simulink model "ENV"  (R2024b)
settings: Solver=FixedStepDiscrete  StartTime=0.0  StopTime=1  FixedStep=0.001  RelTol=1e-3  EnableMultiTasking=on
libraries: stm32blockslib x92, canmsglib x40, simulink x7, stm32f4xxblockslib x6
(part 2 of 5)

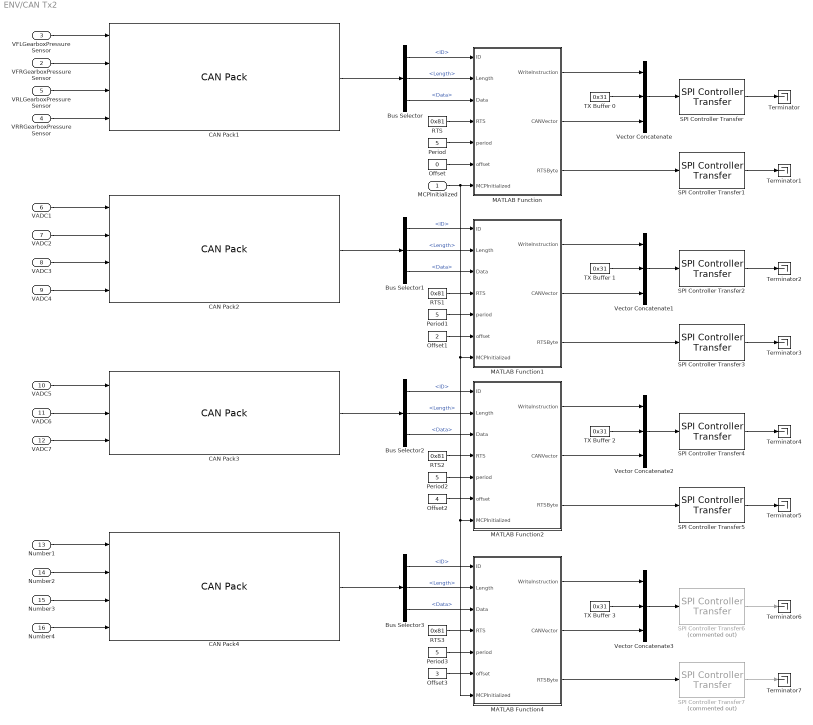
== system ENV/CAN Tx2 ==
  MCPInitialized : Inport
  VFRGearboxPressureSensor : Inport  Port=2
  VFLGearboxPressureSensor : Inport  Port=3
  VRRGearboxPressureSensor : Inport  Port=4
  VRLGearboxPressureSensor : Inport  Port=5
  VADC1 : Inport  Port=6
  VADC2 : Inport  Port=7
  VADC3 : Inport  Port=8
  VADC4 : Inport  Port=9
  VADC5 : Inport  Port=10
  VADC6 : Inport  Port=11
  VADC7 : Inport  Port=12
  Number1 : Inport  Port=13
  Number2 : Inport  Port=14
  Number3 : Inport  Port=15
  Number4 : Inport  Port=16
  Bus Selector{,1..3} (4 alike) : BusSelector  OutputSignals=ID,Length,Data
  CAN Pack1 : canmsglib/CAN Pack  CANdbFile=C:\Users\oxbro\Documents\STM32CustomProjects\PDUSTM32\ADCTest.dbc  MsgList=GearboxPressures  MsgName=GearboxPressures  MsgIDType=Standard (11-bit identifier)  MsgIdentifier=105  CANIDInput=off  MsgLength=8  Remote=off  ApplyMinMax=off  BusOutput=on  SignalInfo={'VFLGearboxPressureSensor','0','12','LE','unsigned','Standard','0','0.0012211','0','0','5.0004';'VFRGearboxPressureSensor','16','12','LE','unsigned','Standard','0','0.0012211','0','0','5.0004';'VRLGearboxPressureSensor','32','12','LE','unsigned','Standard','0','0.0012211','0','0','5.0004';'VRRGearboxPressureSensor','48','12','LE','unsigned','Standard','0','0.0012211','0','0','5.0004'}
      settings: LibrarySourceBlock=stmutilitieslib/CAN Pack  DataFormat=CANdb specified signals
  CAN Pack2 : canmsglib/CAN Pack  CANdbFile=C:\Users\oxbro\Documents\STM32CustomProjects\PDUSTM32\ADCTest.dbc  MsgList=ADCs1  MsgName=ADCs1  MsgIDType=Standard (11-bit identifier)  MsgIdentifier=5  CANIDInput=off  MsgLength=8  Remote=off  ApplyMinMax=off  BusOutput=on  SignalInfo={'VADC1','0','16','LE','unsigned','Standard','0','5.04e-05','0','0','3.303';'VADC2','16','16','LE','unsigned','Standard','0','5.04e-05','0','0','3.303';'VADC3','32','16','LE','unsigned','Standard','0','5.04e-05','0','0','3.303';'VADC4','48','16','LE','unsigned','Standard','0','5.04e-05','0','0','3.303'}
      settings: LibrarySourceBlock=stmutilitieslib/CAN Pack  DataFormat=CANdb specified signals
  CAN Pack3 : canmsglib/CAN Pack  CANdbFile=C:\Users\oxbro\Documents\STM32CustomProjects\PDUSTM32\ADCTest.dbc  MsgList=ADCs2  MsgName=ADCs2  MsgIDType=Standard (11-bit identifier)  MsgIdentifier=66  CANIDInput=off  MsgLength=6  Remote=off  ApplyMinMax=off  BusOutput=on  SignalInfo={'VADC5','0','16','LE','unsigned','Standard','0','5.04e-05','0','0','3.303';'VADC6','16','16','LE','unsigned','Standard','0','5.04e-05','0','0','3.303';'VLVSystem','32','16','LE','unsigned','Standard','0','0.00046327','0','0','30.3604'}
      settings: LibrarySourceBlock=stmutilitieslib/CAN Pack  DataFormat=CANdb specified signals
  CAN Pack4 : canmsglib/CAN Pack  CANdbFile=C:\Users\oxbro\Documents\STM32CustomProjects\PDUSTM32\ADCTest.dbc  MsgList=Numbers  MsgName=Numbers  MsgIDType=Standard (11-bit identifier)  MsgIdentifier=0  CANIDInput=off  MsgLength=8  Remote=off  ApplyMinMax=off  BusOutput=on  SignalInfo={'Number1','0','16','LE','signed','Standard','0','1','0','-32768','32767';'Number2','16','16','LE','signed','Standard','0','1','0','-32768','32767';'Number3','32','16','LE','signed','Standard','0','1','0','-32768','32767';'Number4','48','16','LE','signed','Standard','0','1','0','-32768','32767'}
      settings: LibrarySourceBlock=stmutilitieslib/CAN Pack  DataFormat=CANdb specified signals
  MATLAB Function : MATLAB Function  TreatAsAtomicUnit=on
  MATLAB Function1 : MATLAB Function  TreatAsAtomicUnit=on
  MATLAB Function2 : MATLAB Function  TreatAsAtomicUnit=on
  MATLAB Function4 : MATLAB Function  TreatAsAtomicUnit=on
  Offset : Constant  Value=0  OutDataTypeStr=uint16  SampleTime=-1
  Offset1 : Constant  Value=2  OutDataTypeStr=uint16  SampleTime=-1
  Offset2 : Constant  Value=4  OutDataTypeStr=uint16  SampleTime=-1
  Offset3 : Constant  Value=3  OutDataTypeStr=uint16  SampleTime=-1
  Period{,1..3} (4 alike) : Constant  Value=5  OutDataTypeStr=uint16  SampleTime=-1
  RTS{,1..3} (4 alike) : Constant  Value=0x81  OutDataTypeStr=uint8  SampleTime=-1
  SPI Controller Transfer : stm32blockslib/SPI Controller Transfer  Priority=1  SPIModuleSelect=SPI1  ClockPolarity=Low  ClockPhase=1 Edge  SPIModule=uint32(0)  Mode=Master  BusSpeed=uint32(1000000)  FirstBitToTransfer=Most significant bit (MSB)  ClockMode=0  BlockFunction=Transfer  EnableRegisterAddress=off  RegisterAddress=0  OutputDataType=uint8  OutputDataLength=1  OutputStatus=off  BlockingMode=off  Timeout=0.01  DataBits=8  UseCustomSSPin=Explicit GPIO calls  ActiveLowSSPin=Active low  Port_Select=GPIOA  Pin=1
      settings: LibrarySourceBlock=stm32h7xxblockslib/SPI Controller Transfer
  SPI Controller Transfer1 : stm32blockslib/SPI Controller Transfer  Priority=2  SPIModuleSelect=SPI1  ClockPolarity=Low  ClockPhase=1 Edge  SPIModule=uint32(0)  Mode=Master  BusSpeed=uint32(1000000)  FirstBitToTransfer=Most significant bit (MSB)  ClockMode=0  BlockFunction=Transfer  EnableRegisterAddress=off  RegisterAddress=0  OutputDataType=uint8  OutputDataLength=1  OutputStatus=off  BlockingMode=off  Timeout=0.01  DataBits=8  UseCustomSSPin=Explicit GPIO calls  ActiveLowSSPin=Active low  Port_Select=GPIOA  Pin=1
      settings: LibrarySourceBlock=stm32h7xxblockslib/SPI Controller Transfer
  SPI Controller Transfer2 : stm32blockslib/SPI Controller Transfer  Priority=1  SPIModuleSelect=SPI1  ClockPolarity=Low  ClockPhase=1 Edge  SPIModule=uint32(0)  Mode=Master  BusSpeed=uint32(1000000)  FirstBitToTransfer=Most significant bit (MSB)  ClockMode=0  BlockFunction=Transfer  EnableRegisterAddress=off  RegisterAddress=0  OutputDataType=uint8  OutputDataLength=1  OutputStatus=off  BlockingMode=off  Timeout=0.01  DataBits=8  UseCustomSSPin=Explicit GPIO calls  ActiveLowSSPin=Active low  Port_Select=GPIOA  Pin=1
      settings: LibrarySourceBlock=stm32h7xxblockslib/SPI Controller Transfer
  SPI Controller Transfer3 : stm32blockslib/SPI Controller Transfer  Priority=2  SPIModuleSelect=SPI1  ClockPolarity=Low  ClockPhase=1 Edge  SPIModule=uint32(0)  Mode=Master  BusSpeed=uint32(1000000)  FirstBitToTransfer=Most significant bit (MSB)  ClockMode=0  BlockFunction=Transfer  EnableRegisterAddress=off  RegisterAddress=0  OutputDataType=uint8  OutputDataLength=1  OutputStatus=off  BlockingMode=off  Timeout=0.01  DataBits=8  UseCustomSSPin=Explicit GPIO calls  ActiveLowSSPin=Active low  Port_Select=GPIOA  Pin=1
      settings: LibrarySourceBlock=stm32h7xxblockslib/SPI Controller Transfer
  SPI Controller Transfer4 : stm32blockslib/SPI Controller Transfer  Priority=1  SPIModuleSelect=SPI1  ClockPolarity=Low  ClockPhase=1 Edge  SPIModule=uint32(0)  Mode=Master  BusSpeed=uint32(1000000)  FirstBitToTransfer=Most significant bit (MSB)  ClockMode=0  BlockFunction=Transfer  EnableRegisterAddress=off  RegisterAddress=0  OutputDataType=uint8  OutputDataLength=1  OutputStatus=off  BlockingMode=off  Timeout=0.01  DataBits=8  UseCustomSSPin=Explicit GPIO calls  ActiveLowSSPin=Active low  Port_Select=GPIOA  Pin=1
      settings: LibrarySourceBlock=stm32h7xxblockslib/SPI Controller Transfer
  SPI Controller Transfer5 : stm32blockslib/SPI Controller Transfer  Priority=2  SPIModuleSelect=SPI1  ClockPolarity=Low  ClockPhase=1 Edge  SPIModule=uint32(0)  Mode=Master  BusSpeed=uint32(1000000)  FirstBitToTransfer=Most significant bit (MSB)  ClockMode=0  BlockFunction=Transfer  EnableRegisterAddress=off  RegisterAddress=0  OutputDataType=uint8  OutputDataLength=1  OutputStatus=off  BlockingMode=off  Timeout=0.01  DataBits=8  UseCustomSSPin=Explicit GPIO calls  ActiveLowSSPin=Active low  Port_Select=GPIOA  Pin=1
      settings: LibrarySourceBlock=stm32h7xxblockslib/SPI Controller Transfer
  SPI Controller Transfer6 : stm32blockslib/SPI Controller Transfer  Priority=1  Commented=on  SPIModuleSelect=SPI1  ClockPolarity=Low  ClockPhase=1 Edge  SPIModule=uint32(0)  Mode=Master  BusSpeed=uint32(1000000)  FirstBitToTransfer=Most significant bit (MSB)  ClockMode=0  BlockFunction=Transfer  EnableRegisterAddress=off  RegisterAddress=0  OutputDataType=uint8  OutputDataLength=1  OutputStatus=off  BlockingMode=off  Timeout=0.01  DataBits=8  UseCustomSSPin=Explicit GPIO calls  ActiveLowSSPin=Active low  Port_Select=GPIOA  Pin=1
      settings: LibrarySourceBlock=stm32h7xxblockslib/SPI Controller Transfer
  SPI Controller Transfer7 : stm32blockslib/SPI Controller Transfer  Priority=2  Commented=on  SPIModuleSelect=SPI1  ClockPolarity=Low  ClockPhase=1 Edge  SPIModule=uint32(0)  Mode=Master  BusSpeed=uint32(1000000)  FirstBitToTransfer=Most significant bit (MSB)  ClockMode=0  BlockFunction=Transfer  EnableRegisterAddress=off  RegisterAddress=0  OutputDataType=uint8  OutputDataLength=1  OutputStatus=off  BlockingMode=off  Timeout=0.01  DataBits=8  UseCustomSSPin=Explicit GPIO calls  ActiveLowSSPin=Active low  Port_Select=GPIOA  Pin=1
      settings: LibrarySourceBlock=stm32h7xxblockslib/SPI Controller Transfer
  TX Buffer {0..3} (4 alike) : Constant  Value=0x31  OutDataTypeStr=uint8  SampleTime=-1
  Terminator{,1..7} (8 alike) : Terminator
  Vector Concatenate{,1..3} (4 alike) : Concatenate  NumInputs=3
  wires:
  SPI Controller Transfer/1 -> Terminator/1
  MATLAB Function/1(WriteInstruction) -> Vector Concatenate/1
  RTS/1 -> MATLAB Function/4(RTS)
  MATLAB Function/2(CANVector) -> Vector Concatenate/3
  SPI Controller Transfer1/1 -> Terminator1/1
  Bus Selector/1 -> MATLAB Function/1(ID)  "<ID>"
  Vector Concatenate/1 -> SPI Controller Transfer/1
  TX Buffer 0/1 -> Vector Concatenate/2
  MATLAB Function/3(RTSByte) -> SPI Controller Transfer1/1
  Bus Selector/2 -> MATLAB Function/2(Length)  "<Length>"
  Bus Selector/3 -> MATLAB Function/3(Data)  "<Data>"
  CAN Pack1/1 -> Bus Selector/1
  Period/1 -> MATLAB Function/5(period)
  Offset/1 -> MATLAB Function/6(offset)
  VRLGearboxPressureSensor/1 -> CAN Pack1/3
  VRRGearboxPressureSensor/1 -> CAN Pack1/4
  VFRGearboxPressureSensor/1 -> CAN Pack1/2
  VFLGearboxPressureSensor/1 -> CAN Pack1/1
  SPI Controller Transfer2/1 -> Terminator2/1
  SPI Controller Transfer3/1 -> Terminator3/1
  RTS1/1 -> MATLAB Function1/4(RTS)
  MATLAB Function1/2(CANVector) -> Vector Concatenate1/3
  Bus Selector1/3 -> MATLAB Function1/3(Data)  "<Data>"
  Period1/1 -> MATLAB Function1/5(period)
  Bus Selector1/2 -> MATLAB Function1/2(Length)  "<Length>"
  Offset1/1 -> MATLAB Function1/6(offset)
  CAN Pack2/1 -> Bus Selector1/1
  Bus Selector1/1 -> MATLAB Function1/1(ID)  "<ID>"
  MATLAB Function1/3(RTSByte) -> SPI Controller Transfer3/1
  Vector Concatenate1/1 -> SPI Controller Transfer2/1
  MATLAB Function1/1(WriteInstruction) -> Vector Concatenate1/1
  TX Buffer 1/1 -> Vector Concatenate1/2
  SPI Controller Transfer4/1 -> Terminator4/1
  SPI Controller Transfer5/1 -> Terminator5/1
  RTS2/1 -> MATLAB Function2/4(RTS)
  MATLAB Function2/2(CANVector) -> Vector Concatenate2/3
  Bus Selector2/3 -> MATLAB Function2/3(Data)  "<Data>"
  Period2/1 -> MATLAB Function2/5(period)
  Bus Selector2/2 -> MATLAB Function2/2(Length)  "<Length>"
  Offset2/1 -> MATLAB Function2/6(offset)
  CAN Pack3/1 -> Bus Selector2/1
  Bus Selector2/1 -> MATLAB Function2/1(ID)  "<ID>"
  MATLAB Function2/3(RTSByte) -> SPI Controller Transfer5/1
  Vector Concatenate2/1 -> SPI Controller Transfer4/1
  MATLAB Function2/1(WriteInstruction) -> Vector Concatenate2/1
  TX Buffer 2/1 -> Vector Concatenate2/2
  VADC1/1 -> CAN Pack2/1
  VADC2/1 -> CAN Pack2/2
  VADC3/1 -> CAN Pack2/3
  VADC4/1 -> CAN Pack2/4
  VADC5/1 -> CAN Pack3/1
  VADC6/1 -> CAN Pack3/2
  VADC7/1 -> CAN Pack3/3
  Period3/1 -> MATLAB Function4/5(period)
  Vector Concatenate3/1 -> SPI Controller Transfer6/1
  Offset3/1 -> MATLAB Function4/6(offset)
  Number1/1 -> CAN Pack4/1
  MATLAB Function4/3(RTSByte) -> SPI Controller Transfer7/1
  Number4/1 -> CAN Pack4/4
  MCPInitialized/1 -> MATLAB Function4/7(MCPInitialized), MATLAB Function2/7(MCPInitialized), MATLAB Function1/7(MCPInitialized), MATLAB Function/7(MCPInitialized)
  MATLAB Function4/2(CANVector) -> Vector Concatenate3/3
  Number3/1 -> CAN Pack4/3
  Bus Selector3/3 -> MATLAB Function4/3(Data)  "<Data>"
  Number2/1 -> CAN Pack4/2
  CAN Pack4/1 -> Bus Selector3/1
  Bus Selector3/1 -> MATLAB Function4/1(ID)  "<ID>"
  MATLAB Function4/1(WriteInstruction) -> Vector Concatenate3/1
  TX Buffer 3/1 -> Vector Concatenate3/2
  SPI Controller Transfer6/1 -> Terminator6/1
  SPI Controller Transfer7/1 -> Terminator7/1
  Bus Selector3/2 -> MATLAB Function4/2(Length)  "<Length>"
  RTS3/1 -> MATLAB Function4/4(RTS)

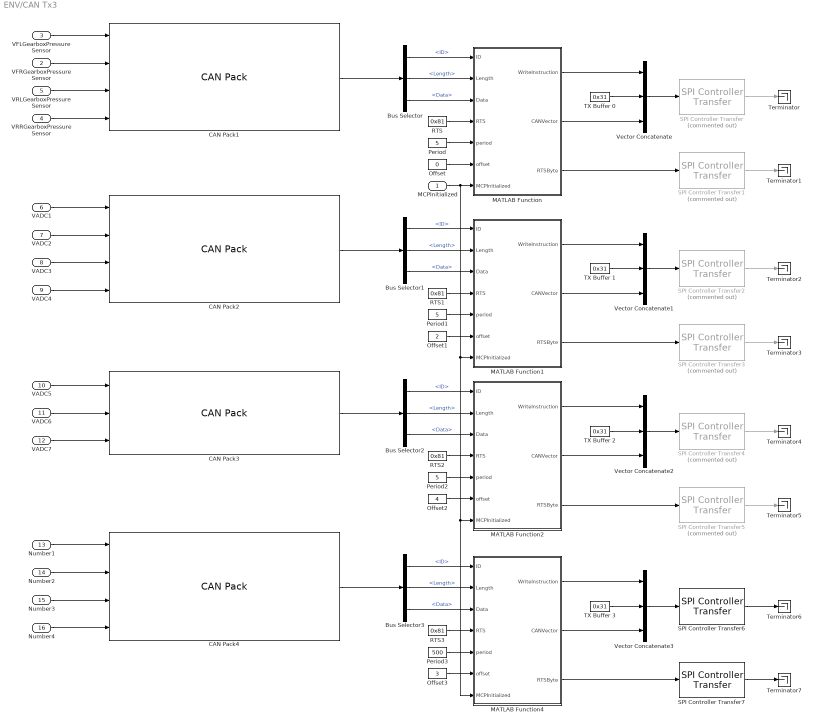
== system ENV/CAN Tx3 ==
  MCPInitialized : Inport
  VFRGearboxPressureSensor : Inport  Port=2
  VFLGearboxPressureSensor : Inport  Port=3
  VRRGearboxPressureSensor : Inport  Port=4
  VRLGearboxPressureSensor : Inport  Port=5
  VADC1 : Inport  Port=6
  VADC2 : Inport  Port=7
  VADC3 : Inport  Port=8
  VADC4 : Inport  Port=9
  VADC5 : Inport  Port=10
  VADC6 : Inport  Port=11
  VADC7 : Inport  Port=12
  Number1 : Inport  Port=13
  Number2 : Inport  Port=14
  Number3 : Inport  Port=15
  Number4 : Inport  Port=16
  Bus Selector{,1..3} (4 alike) : BusSelector  OutputSignals=ID,Length,Data
  CAN Pack1 : canmsglib/CAN Pack  CANdbFile=C:\Users\oxbro\Documents\STM32CustomProjects\PDUSTM32\ADCTest.dbc  MsgList=GearboxPressures  MsgName=GearboxPressures  MsgIDType=Standard (11-bit identifier)  MsgIdentifier=105  CANIDInput=off  MsgLength=8  Remote=off  ApplyMinMax=off  BusOutput=on  SignalInfo={'VFLGearboxPressureSensor','0','12','LE','unsigned','Standard','0','0.0012211','0','0','5.0004';'VFRGearboxPressureSensor','16','12','LE','unsigned','Standard','0','0.0012211','0','0','5.0004';'VRLGearboxPressureSensor','32','12','LE','unsigned','Standard','0','0.0012211','0','0','5.0004';'VRRGearboxPressureSensor','48','12','LE','unsigned','Standard','0','0.0012211','0','0','5.0004'}
      settings: LibrarySourceBlock=stmutilitieslib/CAN Pack  DataFormat=CANdb specified signals
  CAN Pack2 : canmsglib/CAN Pack  CANdbFile=C:\Users\oxbro\Documents\STM32CustomProjects\PDUSTM32\ADCTest.dbc  MsgList=ADCs1  MsgName=ADCs1  MsgIDType=Standard (11-bit identifier)  MsgIdentifier=5  CANIDInput=off  MsgLength=8  Remote=off  ApplyMinMax=off  BusOutput=on  SignalInfo={'VADC1','0','16','LE','unsigned','Standard','0','5.04e-05','0','0','3.303';'VADC2','16','16','LE','unsigned','Standard','0','5.04e-05','0','0','3.303';'VADC3','32','16','LE','unsigned','Standard','0','5.04e-05','0','0','3.303';'VADC4','48','16','LE','unsigned','Standard','0','5.04e-05','0','0','3.303'}
      settings: LibrarySourceBlock=stmutilitieslib/CAN Pack  DataFormat=CANdb specified signals
  CAN Pack3 : canmsglib/CAN Pack  CANdbFile=C:\Users\oxbro\Documents\STM32CustomProjects\PDUSTM32\ADCTest.dbc  MsgList=ADCs2  MsgName=ADCs2  MsgIDType=Standard (11-bit identifier)  MsgIdentifier=66  CANIDInput=off  MsgLength=6  Remote=off  ApplyMinMax=off  BusOutput=on  SignalInfo={'VADC5','0','16','LE','unsigned','Standard','0','5.04e-05','0','0','3.303';'VADC6','16','16','LE','unsigned','Standard','0','5.04e-05','0','0','3.303';'VLVSystem','32','16','LE','unsigned','Standard','0','0.00046327','0','0','30.3604'}
      settings: LibrarySourceBlock=stmutilitieslib/CAN Pack  DataFormat=CANdb specified signals
  CAN Pack4 : canmsglib/CAN Pack  CANdbFile=C:\Users\oxbro\Documents\STM32CustomProjects\PDUSTM32\ADCTest.dbc  MsgList=Numbers  MsgName=Numbers  MsgIDType=Standard (11-bit identifier)  MsgIdentifier=0  CANIDInput=off  MsgLength=8  Remote=off  ApplyMinMax=off  BusOutput=on  SignalInfo={'Number1','0','16','LE','signed','Standard','0','1','0','-32768','32767';'Number2','16','16','LE','signed','Standard','0','1','0','-32768','32767';'Number3','32','16','LE','signed','Standard','0','1','0','-32768','32767';'Number4','48','16','LE','signed','Standard','0','1','0','-32768','32767'}
      settings: LibrarySourceBlock=stmutilitieslib/CAN Pack  DataFormat=CANdb specified signals
  MATLAB Function : MATLAB Function  TreatAsAtomicUnit=on
  MATLAB Function1 : MATLAB Function  TreatAsAtomicUnit=on
  MATLAB Function2 : MATLAB Function  TreatAsAtomicUnit=on
  MATLAB Function4 : MATLAB Function  TreatAsAtomicUnit=on
  Offset : Constant  Value=0  OutDataTypeStr=uint16  SampleTime=-1
  Offset1 : Constant  Value=2  OutDataTypeStr=uint16  SampleTime=-1
  Offset2 : Constant  Value=4  OutDataTypeStr=uint16  SampleTime=-1
  Offset3 : Constant  Value=3  OutDataTypeStr=uint16  SampleTime=-1
  Period : Constant  Value=5  OutDataTypeStr=uint16  SampleTime=-1
  Period1 : Constant  Value=5  OutDataTypeStr=uint16  SampleTime=-1
  Period2 : Constant  Value=5  OutDataTypeStr=uint16  SampleTime=-1
  Period3 : Constant  Value=500  OutDataTypeStr=uint16  SampleTime=-1
  RTS{,1..3} (4 alike) : Constant  Value=0x81  OutDataTypeStr=uint8  SampleTime=-1
  SPI Controller Transfer : stm32blockslib/SPI Controller Transfer  Priority=1  Commented=on  SPIModuleSelect=SPI1  ClockPolarity=Low  ClockPhase=1 Edge  SPIModule=uint32(0)  Mode=Master  BusSpeed=uint32(1000000)  FirstBitToTransfer=Most significant bit (MSB)  ClockMode=0  BlockFunction=Transfer  EnableRegisterAddress=off  RegisterAddress=0  OutputDataType=uint8  OutputDataLength=1  OutputStatus=off  BlockingMode=off  Timeout=0.01  DataBits=8  UseCustomSSPin=Explicit GPIO calls  ActiveLowSSPin=Active low  Port_Select=GPIOA  Pin=1
      settings: LibrarySourceBlock=stm32h7xxblockslib/SPI Controller Transfer
  SPI Controller Transfer1 : stm32blockslib/SPI Controller Transfer  Priority=2  Commented=on  SPIModuleSelect=SPI1  ClockPolarity=Low  ClockPhase=1 Edge  SPIModule=uint32(0)  Mode=Master  BusSpeed=uint32(1000000)  FirstBitToTransfer=Most significant bit (MSB)  ClockMode=0  BlockFunction=Transfer  EnableRegisterAddress=off  RegisterAddress=0  OutputDataType=uint8  OutputDataLength=1  OutputStatus=off  BlockingMode=off  Timeout=0.01  DataBits=8  UseCustomSSPin=Explicit GPIO calls  ActiveLowSSPin=Active low  Port_Select=GPIOA  Pin=1
      settings: LibrarySourceBlock=stm32h7xxblockslib/SPI Controller Transfer
  SPI Controller Transfer2 : stm32blockslib/SPI Controller Transfer  Priority=1  Commented=on  SPIModuleSelect=SPI1  ClockPolarity=Low  ClockPhase=1 Edge  SPIModule=uint32(0)  Mode=Master  BusSpeed=uint32(1000000)  FirstBitToTransfer=Most significant bit (MSB)  ClockMode=0  BlockFunction=Transfer  EnableRegisterAddress=off  RegisterAddress=0  OutputDataType=uint8  OutputDataLength=1  OutputStatus=off  BlockingMode=off  Timeout=0.01  DataBits=8  UseCustomSSPin=Explicit GPIO calls  ActiveLowSSPin=Active low  Port_Select=GPIOA  Pin=1
      settings: LibrarySourceBlock=stm32h7xxblockslib/SPI Controller Transfer
  SPI Controller Transfer3 : stm32blockslib/SPI Controller Transfer  Priority=2  Commented=on  SPIModuleSelect=SPI1  ClockPolarity=Low  ClockPhase=1 Edge  SPIModule=uint32(0)  Mode=Master  BusSpeed=uint32(1000000)  FirstBitToTransfer=Most significant bit (MSB)  ClockMode=0  BlockFunction=Transfer  EnableRegisterAddress=off  RegisterAddress=0  OutputDataType=uint8  OutputDataLength=1  OutputStatus=off  BlockingMode=off  Timeout=0.01  DataBits=8  UseCustomSSPin=Explicit GPIO calls  ActiveLowSSPin=Active low  Port_Select=GPIOA  Pin=1
      settings: LibrarySourceBlock=stm32h7xxblockslib/SPI Controller Transfer
  SPI Controller Transfer4 : stm32blockslib/SPI Controller Transfer  Priority=1  Commented=on  SPIModuleSelect=SPI1  ClockPolarity=Low  ClockPhase=1 Edge  SPIModule=uint32(0)  Mode=Master  BusSpeed=uint32(1000000)  FirstBitToTransfer=Most significant bit (MSB)  ClockMode=0  BlockFunction=Transfer  EnableRegisterAddress=off  RegisterAddress=0  OutputDataType=uint8  OutputDataLength=1  OutputStatus=off  BlockingMode=off  Timeout=0.01  DataBits=8  UseCustomSSPin=Explicit GPIO calls  ActiveLowSSPin=Active low  Port_Select=GPIOA  Pin=1
      settings: LibrarySourceBlock=stm32h7xxblockslib/SPI Controller Transfer
  SPI Controller Transfer5 : stm32blockslib/SPI Controller Transfer  Priority=2  Commented=on  SPIModuleSelect=SPI1  ClockPolarity=Low  ClockPhase=1 Edge  SPIModule=uint32(0)  Mode=Master  BusSpeed=uint32(1000000)  FirstBitToTransfer=Most significant bit (MSB)  ClockMode=0  BlockFunction=Transfer  EnableRegisterAddress=off  RegisterAddress=0  OutputDataType=uint8  OutputDataLength=1  OutputStatus=off  BlockingMode=off  Timeout=0.01  DataBits=8  UseCustomSSPin=Explicit GPIO calls  ActiveLowSSPin=Active low  Port_Select=GPIOA  Pin=1
      settings: LibrarySourceBlock=stm32h7xxblockslib/SPI Controller Transfer
  SPI Controller Transfer6 : stm32blockslib/SPI Controller Transfer  Priority=1  SPIModuleSelect=SPI1  ClockPolarity=Low  ClockPhase=1 Edge  SPIModule=uint32(0)  Mode=Master  BusSpeed=uint32(1000000)  FirstBitToTransfer=Most significant bit (MSB)  ClockMode=0  BlockFunction=Transfer  EnableRegisterAddress=off  RegisterAddress=0  OutputDataType=uint8  OutputDataLength=1  OutputStatus=off  BlockingMode=off  Timeout=0.01  DataBits=8  UseCustomSSPin=Explicit GPIO calls  ActiveLowSSPin=Active low  Port_Select=GPIOC  Pin=5
      settings: LibrarySourceBlock=stm32h7xxblockslib/SPI Controller Transfer
  SPI Controller Transfer7 : stm32blockslib/SPI Controller Transfer  Priority=2  SPIModuleSelect=SPI1  ClockPolarity=Low  ClockPhase=1 Edge  SPIModule=uint32(0)  Mode=Master  BusSpeed=uint32(1000000)  FirstBitToTransfer=Most significant bit (MSB)  ClockMode=0  BlockFunction=Transfer  EnableRegisterAddress=off  RegisterAddress=0  OutputDataType=uint8  OutputDataLength=1  OutputStatus=off  BlockingMode=off  Timeout=0.01  DataBits=8  UseCustomSSPin=Explicit GPIO calls  ActiveLowSSPin=Active low  Port_Select=GPIOC  Pin=5
      settings: LibrarySourceBlock=stm32h7xxblockslib/SPI Controller Transfer
  TX Buffer {0..3} (4 alike) : Constant  Value=0x31  OutDataTypeStr=uint8  SampleTime=-1
  Terminator{,1..7} (8 alike) : Terminator
  Vector Concatenate{,1..3} (4 alike) : Concatenate  NumInputs=3
  wires:
  SPI Controller Transfer/1 -> Terminator/1
  MATLAB Function/1(WriteInstruction) -> Vector Concatenate/1
  RTS/1 -> MATLAB Function/4(RTS)
  MATLAB Function/2(CANVector) -> Vector Concatenate/3
  SPI Controller Transfer1/1 -> Terminator1/1
  Bus Selector/1 -> MATLAB Function/1(ID)  "<ID>"
  Vector Concatenate/1 -> SPI Controller Transfer/1
  TX Buffer 0/1 -> Vector Concatenate/2
  MATLAB Function/3(RTSByte) -> SPI Controller Transfer1/1
  Bus Selector/2 -> MATLAB Function/2(Length)  "<Length>"
  Bus Selector/3 -> MATLAB Function/3(Data)  "<Data>"
  CAN Pack1/1 -> Bus Selector/1
  Period/1 -> MATLAB Function/5(period)
  Offset/1 -> MATLAB Function/6(offset)
  VRLGearboxPressureSensor/1 -> CAN Pack1/3
  VRRGearboxPressureSensor/1 -> CAN Pack1/4
  VFRGearboxPressureSensor/1 -> CAN Pack1/2
  VFLGearboxPressureSensor/1 -> CAN Pack1/1
  SPI Controller Transfer2/1 -> Terminator2/1
  SPI Controller Transfer3/1 -> Terminator3/1
  RTS1/1 -> MATLAB Function1/4(RTS)
  MATLAB Function1/2(CANVector) -> Vector Concatenate1/3
  Bus Selector1/3 -> MATLAB Function1/3(Data)  "<Data>"
  Period1/1 -> MATLAB Function1/5(period)
  Bus Selector1/2 -> MATLAB Function1/2(Length)  "<Length>"
  Offset1/1 -> MATLAB Function1/6(offset)
  CAN Pack2/1 -> Bus Selector1/1
  Bus Selector1/1 -> MATLAB Function1/1(ID)  "<ID>"
  MATLAB Function1/3(RTSByte) -> SPI Controller Transfer3/1
  Vector Concatenate1/1 -> SPI Controller Transfer2/1
  MATLAB Function1/1(WriteInstruction) -> Vector Concatenate1/1
  TX Buffer 1/1 -> Vector Concatenate1/2
  SPI Controller Transfer4/1 -> Terminator4/1
  SPI Controller Transfer5/1 -> Terminator5/1
  RTS2/1 -> MATLAB Function2/4(RTS)
  MATLAB Function2/2(CANVector) -> Vector Concatenate2/3
  Bus Selector2/3 -> MATLAB Function2/3(Data)  "<Data>"
  Period2/1 -> MATLAB Function2/5(period)
  Bus Selector2/2 -> MATLAB Function2/2(Length)  "<Length>"
  Offset2/1 -> MATLAB Function2/6(offset)
  CAN Pack3/1 -> Bus Selector2/1
  Bus Selector2/1 -> MATLAB Function2/1(ID)  "<ID>"
  MATLAB Function2/3(RTSByte) -> SPI Controller Transfer5/1
  Vector Concatenate2/1 -> SPI Controller Transfer4/1
  MATLAB Function2/1(WriteInstruction) -> Vector Concatenate2/1
  TX Buffer 2/1 -> Vector Concatenate2/2
  VADC1/1 -> CAN Pack2/1
  VADC2/1 -> CAN Pack2/2
  VADC3/1 -> CAN Pack2/3
  VADC4/1 -> CAN Pack2/4
  VADC5/1 -> CAN Pack3/1
  VADC6/1 -> CAN Pack3/2
  VADC7/1 -> CAN Pack3/3
  Period3/1 -> MATLAB Function4/5(period)
  Vector Concatenate3/1 -> SPI Controller Transfer6/1
  Offset3/1 -> MATLAB Function4/6(offset)
  Number1/1 -> CAN Pack4/1
  MATLAB Function4/3(RTSByte) -> SPI Controller Transfer7/1
  Number4/1 -> CAN Pack4/4
  MCPInitialized/1 -> MATLAB Function4/7(MCPInitialized), MATLAB Function2/7(MCPInitialized), MATLAB Function1/7(MCPInitialized), MATLAB Function/7(MCPInitialized)
  MATLAB Function4/2(CANVector) -> Vector Concatenate3/3
  Number3/1 -> CAN Pack4/3
  Bus Selector3/3 -> MATLAB Function4/3(Data)  "<Data>"
  Number2/1 -> CAN Pack4/2
  CAN Pack4/1 -> Bus Selector3/1
  Bus Selector3/1 -> MATLAB Function4/1(ID)  "<ID>"
  MATLAB Function4/1(WriteInstruction) -> Vector Concatenate3/1
  TX Buffer 3/1 -> Vector Concatenate3/2
  SPI Controller Transfer6/1 -> Terminator6/1
  SPI Controller Transfer7/1 -> Terminator7/1
  Bus Selector3/2 -> MATLAB Function4/2(Length)  "<Length>"
  RTS3/1 -> MATLAB Function4/4(RTS)

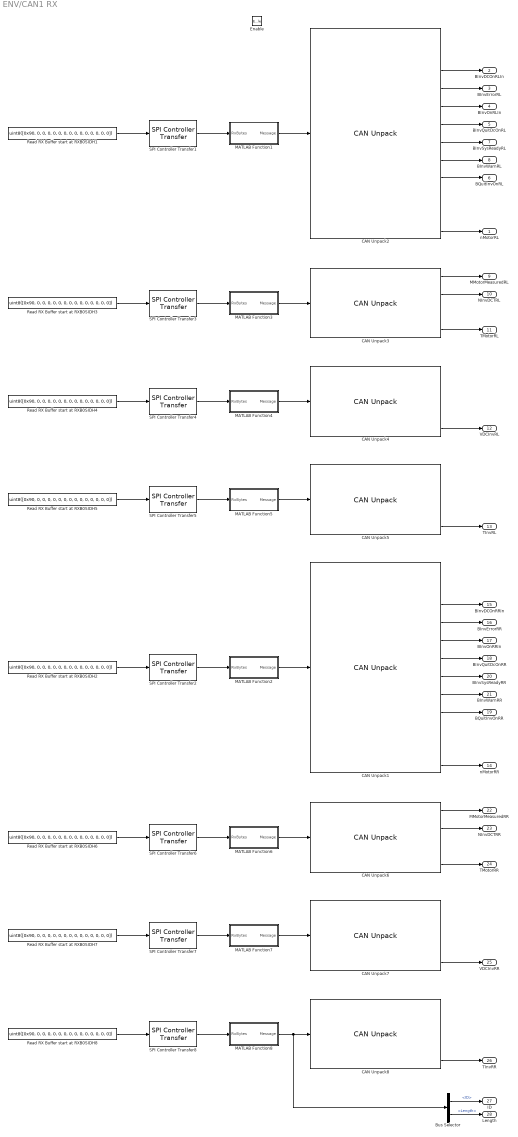
== system ENV/CAN1 RX ==
  Enable : EnablePort
  Bus Selector : BusSelector  OutputSignals=ID,Length
  CAN Unpack1 : canmsglib/CAN Unpack  CANdbFile=C:\Users\Will\Desktop\OBR\Embedded\VCUSTM32\Controls\CAN\Inverters\26.06.18_CAN1.dbc  MsgList=INV3_Send_1  MsgName=INV3_Send_1  MsgIDType=Standard (11-bit identifier)  MsgIdentifier=644  MsgLength=8  SignalInfo={'AMK_bDerating','47','1','LE','unsigned','Standard','0','1','0','0','1';'AMK_bReserve','32','8','LE','signed','Standard','0','1','0','-128','127';'BInvDCOnRRIn','44','1','LE','unsigned','Standard','0','1','0','0','1';'BInvErrorRR','41','1','LE','unsigned','Standard','0','1','0','0','1';'BInvOnRRIn','46','1','LE','unsigned','Standard','0','1','0','0','1';'BInvQuitDcOnRR','43','1','LE','unsigned','Standard','0','1','0','0','1';'BInvSysReadyRR','40','1','LE','unsigned','Standard','0','1','0','0','1';'BInvWarnRR','42','1','LE','unsigned','Standard','0','1','0','0','1';'BQuitInvOnRR','45','1','LE','unsigned','Standard','0','1','0','0','1';'Checksum','16','16','LE','unsigned','Standard','0','1','0','0','65535';'Message_Counter','0','16','LE','unsigned','Standard','0','1','0','0','65535';'nMotorRR','48','16','LE','signed','Standard','0','1','0','-32768','32767'}  IDPort=off  TimestampPort=off  ErrorPort=off  RemotePort=off  LengthPort=off  StatusPort=off  ApplyMinMax=off
      settings: LibrarySourceBlock=stmutilitieslib/CAN Unpack  DataFormat=CANdb specified signals
  CAN Unpack2 : canmsglib/CAN Unpack  CANdbFile=C:\Users\Will\Desktop\OBR\Embedded\VCUSTM32\Controls\CAN\Inverters\26.06.18_CAN1.dbc  MsgList=INV1_Send_1  MsgName=INV1_Send_1  MsgIDType=Standard (11-bit identifier)  MsgIdentifier=643  MsgLength=8  SignalInfo={'AMK_bDerating','47','1','LE','unsigned','Standard','0','1','0','0','1';'AMK_bReserve','32','8','LE','signed','Standard','0','1','0','-128','127';'BInvDCOnRLIn','44','1','LE','unsigned','Standard','0','1','0','0','1';'BInvErrorRL','41','1','LE','unsigned','Standard','0','1','0','0','1';'BInvOnRLIn','46','1','LE','unsigned','Standard','0','1','0','0','1';'BInvQuitDcOnRL','43','1','LE','unsigned','Standard','0','1','0','0','1';'BInvSysReadyRL','40','1','LE','unsigned','Standard','0','1','0','0','1';'BInvWarnRL','42','1','LE','unsigned','Standard','0','1','0','0','1';'BQuitInvOnRL','45','1','LE','unsigned','Standard','0','1','0','0','1';'Checksum','16','16','LE','unsigned','Standard','0','1','0','0','65535';'Message_Counter','0','16','LE','unsigned','Standard','0','1','0','0','65535';'nMotorRL','48','16','LE','signed','Standard','0','1','0','-32768','32767'}  IDPort=off  TimestampPort=off  ErrorPort=off  RemotePort=off  LengthPort=off  StatusPort=off  ApplyMinMax=off
      settings: LibrarySourceBlock=stmutilitieslib/CAN Unpack  DataFormat=CANdb specified signals
  CAN Unpack3 : canmsglib/CAN Unpack  CANdbFile=C:\Users\Will\Desktop\OBR\Embedded\VCUSTM32\Controls\CAN\Inverters\26.06.18_CAN1.dbc  MsgList=INV1_Send_2  MsgName=INV1_Send_2  MsgIDType=Standard (11-bit identifier)  MsgIdentifier=645  MsgLength=8  SignalInfo={'MMotorMeasuredRL','16','16','LE','signed','Standard','0','1','0','-32768','32767';'NInvDTCRL','32','16','LE','signed','Standard','0','1','0','-32768','32767';'NInvErrorInfoRL1','48','16','LE','signed','Standard','0','1','0','-32768','32767';'TMotorRL','0','16','LE','signed','Standard','0','0.1','0','-3276.8','3276.7'}  IDPort=off  TimestampPort=off  ErrorPort=off  RemotePort=off  LengthPort=off  StatusPort=off  ApplyMinMax=off
      settings: LibrarySourceBlock=stmutilitieslib/CAN Unpack  DataFormat=CANdb specified signals
  CAN Unpack4 : canmsglib/CAN Unpack  CANdbFile=C:\Users\Will\Desktop\OBR\Embedded\VCUSTM32\Controls\CAN\Inverters\26.06.18_CAN1.dbc  MsgList=INV1_Send_3  MsgName=INV1_Send_3  MsgIDType=Standard (11-bit identifier)  MsgIdentifier=647  MsgLength=8  SignalInfo={'NInvErrorInfoRL2','0','16','LE','signed','Standard','0','1','0','-32768','32767';'NInvErrorInfoRL3','16','16','LE','signed','Standard','0','1','0','-32768','32767';'Raw_Torque_Current','32','16','LE','signed','Standard','0','1','0','-32768','32767';'VDCInvRL','48','16','LE','signed','Standard','0','1','0','-32768','32767'}  IDPort=off  TimestampPort=off  ErrorPort=off  RemotePort=off  LengthPort=off  StatusPort=off  ApplyMinMax=off
      settings: LibrarySourceBlock=stmutilitieslib/CAN Unpack  DataFormat=CANdb specified signals
  CAN Unpack5 : canmsglib/CAN Unpack  CANdbFile=C:\Users\Will\Desktop\OBR\Embedded\VCUSTM32\Controls\CAN\Inverters\26.06.18_CAN1.dbc  MsgList=INV1_Send_4  MsgName=INV1_Send_4  MsgIDType=Standard (11-bit identifier)  MsgIdentifier=649  MsgLength=8  SignalInfo={'Converter_Peak_Current','32','16','LE','signed','Standard','0','1','0','-32768','32767';'Motor_Nomial_Current_IN','48','16','LE','signed','Standard','0','1','0','-32768','32767';'Motor_Peak_Current','16','16','LE','signed','Standard','0','1','0','-32768','32767';'TInvRL','0','16','LE','signed','Standard','0','0.1','0','-3276.8','3276.7'}  IDPort=off  TimestampPort=off  ErrorPort=off  RemotePort=off  LengthPort=off  StatusPort=off  ApplyMinMax=off
      settings: LibrarySourceBlock=stmutilitieslib/CAN Unpack  DataFormat=CANdb specified signals
  CAN Unpack6 : canmsglib/CAN Unpack  CANdbFile=C:\Users\Will\Desktop\OBR\Embedded\VCUSTM32\Controls\CAN\Inverters\26.06.18_CAN1.dbc  MsgList=INV3_Send_2  MsgName=INV3_Send_2  MsgIDType=Standard (11-bit identifier)  MsgIdentifier=646  MsgLength=8  SignalInfo={'MMotorMeasuredRR','16','16','LE','signed','Standard','0','1','0','-32768','32767';'NInvDTCRR','32','16','LE','signed','Standard','0','1','0','-32768','32767';'NInvErrorInfoRR1','48','16','LE','signed','Standard','0','1','0','-32768','32767';'TMotorRR','0','16','LE','signed','Standard','0','0.1','0','-3276.8','3276.7'}  IDPort=off  TimestampPort=off  ErrorPort=off  RemotePort=off  LengthPort=off  StatusPort=off  ApplyMinMax=off
      settings: LibrarySourceBlock=stmutilitieslib/CAN Unpack  DataFormat=CANdb specified signals
  CAN Unpack7 : canmsglib/CAN Unpack  CANdbFile=C:\Users\Will\Desktop\OBR\Embedded\VCUSTM32\Controls\CAN\Inverters\26.06.18_CAN1.dbc  MsgList=INV3_Send_3  MsgName=INV3_Send_3  MsgIDType=Standard (11-bit identifier)  MsgIdentifier=648  MsgLength=8  SignalInfo={'NInvErrorInfoRR2','0','16','LE','signed','Standard','0','1','0','-32768','32767';'NInvErrorInfoRR3','16','16','LE','signed','Standard','0','1','0','-32768','32767';'Raw_Torque_Current','32','16','LE','signed','Standard','0','1','0','-32768','32767';'VDCInvRR','48','16','LE','signed','Standard','0','1','0','-32768','32767'}  IDPort=off  TimestampPort=off  ErrorPort=off  RemotePort=off  LengthPort=off  StatusPort=off  ApplyMinMax=off
      settings: LibrarySourceBlock=stmutilitieslib/CAN Unpack  DataFormat=CANdb specified signals
  CAN Unpack8 : canmsglib/CAN Unpack  CANdbFile=C:\Users\Will\Desktop\OBR\Embedded\VCUSTM32\Controls\CAN\Inverters\26.06.18_CAN1.dbc  MsgList=INV3_Send_4  MsgName=INV3_Send_4  MsgIDType=Standard (11-bit identifier)  MsgIdentifier=656  MsgLength=8  SignalInfo={'Converter_Peak_Current','32','16','LE','signed','Standard','0','1','0','-32768','32767';'Motor_Nomial_Current_IN','48','16','LE','signed','Standard','0','1','0','-32768','32767';'Motor_Peak_Current','16','16','LE','signed','Standard','0','1','0','-32768','32767';'TInvRR','0','16','LE','signed','Standard','0','0.1','0','-3276.8','3276.7'}  IDPort=off  TimestampPort=off  ErrorPort=off  RemotePort=off  LengthPort=off  StatusPort=off  ApplyMinMax=off
      settings: LibrarySourceBlock=stmutilitieslib/CAN Unpack  DataFormat=CANdb specified signals
  MATLAB Function1 : MATLAB Function  TreatAsAtomicUnit=on
  MATLAB Function2 : MATLAB Function  TreatAsAtomicUnit=on
  MATLAB Function3 : MATLAB Function  TreatAsAtomicUnit=on
  MATLAB Function4 : MATLAB Function  TreatAsAtomicUnit=on
  MATLAB Function5 : MATLAB Function  TreatAsAtomicUnit=on
  MATLAB Function6 : MATLAB Function  TreatAsAtomicUnit=on
  MATLAB Function7 : MATLAB Function  TreatAsAtomicUnit=on
  MATLAB Function8 : MATLAB Function  TreatAsAtomicUnit=on
  Read RX Buffer start at RXB0SIDH{1..8} (8 alike) : Constant  Value=uint8([0x90, 0, 0, 0, 0, 0, 0, 0, 0, 0, 0, 0, 0, 0, 0])
  SPI Controller Transfer{1..8} (8 alike) : stm32blockslib/SPI Controller Transfer  Priority=1  SPIModuleSelect=SPI1  ClockPolarity=Low  ClockPhase=1 Edge  SPIModule=uint32(0)  Mode=Master  BusSpeed=uint32(1000000)  FirstBitToTransfer=Most significant bit (MSB)  ClockMode=0  BlockFunction=Transfer  EnableRegisterAddress=off  RegisterAddress=0  OutputDataType=uint8  OutputDataLength=1  OutputStatus=off  BlockingMode=on  Timeout=0.01  DataBits=8  UseCustomSSPin=Explicit GPIO calls  ActiveLowSSPin=Active low  Port_Select=GPIOB  Pin=1
      settings: LibrarySourceBlock=stm32h7xxblockslib/SPI Controller Transfer
  nMotorRL : Outport  OutDataTypeStr=double
  BInvDCOnRLIn : Outport  Port=2  OutDataTypeStr=boolean
  BInvErrorRL : Outport  Port=3  OutDataTypeStr=boolean
  BInvOnRLIn : Outport  Port=4  OutDataTypeStr=boolean
  BInvQuitDcOnRL : Outport  Port=5  OutDataTypeStr=boolean
  BQuitInvOnRL : Outport  Port=6  OutDataTypeStr=boolean
  BInvSysReadyRL : Outport  Port=7  OutDataTypeStr=boolean
  BInvWarnRL : Outport  Port=8  OutDataTypeStr=boolean
  MMotorMeasuredRL : Outport  Port=9  OutDataTypeStr=double
  NInvDCTRL : Outport  Port=10  OutDataTypeStr=double
  TMotorRL : Outport  Port=11  OutDataTypeStr=double
  VDCInvRL : Outport  Port=12  OutDataTypeStr=double
  TInvRL : Outport  Port=13  OutDataTypeStr=double
  nMotorRR : Outport  Port=14  OutDataTypeStr=double
  BInvDCOnRRIn : Outport  Port=15  OutDataTypeStr=boolean
  BInvErrorRR : Outport  Port=16  OutDataTypeStr=boolean
  BInvOnRRIn : Outport  Port=17  OutDataTypeStr=boolean
  BInvQuitDcOnRR : Outport  Port=18  OutDataTypeStr=boolean
  BQuitInvOnRR : Outport  Port=19  OutDataTypeStr=boolean
  BInvSysReadyRR : Outport  Port=20  OutDataTypeStr=boolean
  BInvWarnRR : Outport  Port=21  OutDataTypeStr=boolean
  MMotorMeasuredRR : Outport  Port=22  OutDataTypeStr=double
  NInvDCTRR : Outport  Port=23  OutDataTypeStr=double
  TMotorRR : Outport  Port=24  OutDataTypeStr=double
  VDCInvRR : Outport  Port=25  OutDataTypeStr=double
  TInvRR : Outport  Port=26  OutDataTypeStr=double
  ID : Outport  Port=27
  Length : Outport  Port=28
  wires:
  Read RX Buffer start at RXB0SIDH1/1 -> SPI Controller Transfer1/1
  SPI Controller Transfer1/1 -> MATLAB Function1/1(RxBytes)
  MATLAB Function1/1(Message) -> CAN Unpack2/1
  CAN Unpack2/3 -> BInvDCOnRLIn/1
  CAN Unpack2/4 -> BInvErrorRL/1
  CAN Unpack2/5 -> BInvOnRLIn/1
  CAN Unpack2/6 -> BInvQuitDcOnRL/1
  CAN Unpack2/9 -> BQuitInvOnRL/1
  CAN Unpack2/8 -> BInvWarnRL/1
  CAN Unpack2/7 -> BInvSysReadyRL/1
  CAN Unpack2/12 -> nMotorRL/1
  CAN Unpack3/4 -> TMotorRL/1
  MATLAB Function3/1(Message) -> CAN Unpack3/1
  SPI Controller Transfer3/1 -> MATLAB Function3/1(RxBytes)
  Read RX Buffer start at RXB0SIDH3/1 -> SPI Controller Transfer3/1
  CAN Unpack3/1 -> MMotorMeasuredRL/1
  CAN Unpack3/2 -> NInvDCTRL/1
  CAN Unpack4/4 -> VDCInvRL/1
  SPI Controller Transfer4/1 -> MATLAB Function4/1(RxBytes)
  MATLAB Function4/1(Message) -> CAN Unpack4/1
  Read RX Buffer start at RXB0SIDH4/1 -> SPI Controller Transfer4/1
  SPI Controller Transfer5/1 -> MATLAB Function5/1(RxBytes)
  CAN Unpack5/4 -> TInvRL/1
  Read RX Buffer start at RXB0SIDH5/1 -> SPI Controller Transfer5/1
  MATLAB Function5/1(Message) -> CAN Unpack5/1
  MATLAB Function8/1(Message) -> CAN Unpack8/1, Bus Selector/1
  Bus Selector/2 -> Length/1  "<Length>"
  Bus Selector/1 -> ID/1  "<ID>"
  CAN Unpack1/6 -> BInvQuitDcOnRR/1
  CAN Unpack1/3 -> BInvDCOnRRIn/1
  CAN Unpack6/4 -> TMotorRR/1
  CAN Unpack1/5 -> BInvOnRRIn/1
  SPI Controller Transfer2/1 -> MATLAB Function2/1(RxBytes)
  MATLAB Function2/1(Message) -> CAN Unpack1/1
  SPI Controller Transfer8/1 -> MATLAB Function8/1(RxBytes)
  CAN Unpack1/8 -> BInvWarnRR/1
  CAN Unpack6/1 -> MMotorMeasuredRR/1
  CAN Unpack1/12 -> nMotorRR/1
  CAN Unpack1/4 -> BInvErrorRR/1
  CAN Unpack1/7 -> BInvSysReadyRR/1
  CAN Unpack1/9 -> BQuitInvOnRR/1
  Read RX Buffer start at RXB0SIDH2/1 -> SPI Controller Transfer2/1
  SPI Controller Transfer7/1 -> MATLAB Function7/1(RxBytes)
  Read RX Buffer start at RXB0SIDH8/1 -> SPI Controller Transfer8/1
  MATLAB Function6/1(Message) -> CAN Unpack6/1
  Read RX Buffer start at RXB0SIDH7/1 -> SPI Controller Transfer7/1
  CAN Unpack6/2 -> NInvDCTRR/1
  SPI Controller Transfer6/1 -> MATLAB Function6/1(RxBytes)
  MATLAB Function7/1(Message) -> CAN Unpack7/1
  Read RX Buffer start at RXB0SIDH6/1 -> SPI Controller Transfer6/1
  CAN Unpack7/4 -> VDCInvRR/1
  CAN Unpack8/4 -> TInvRR/1

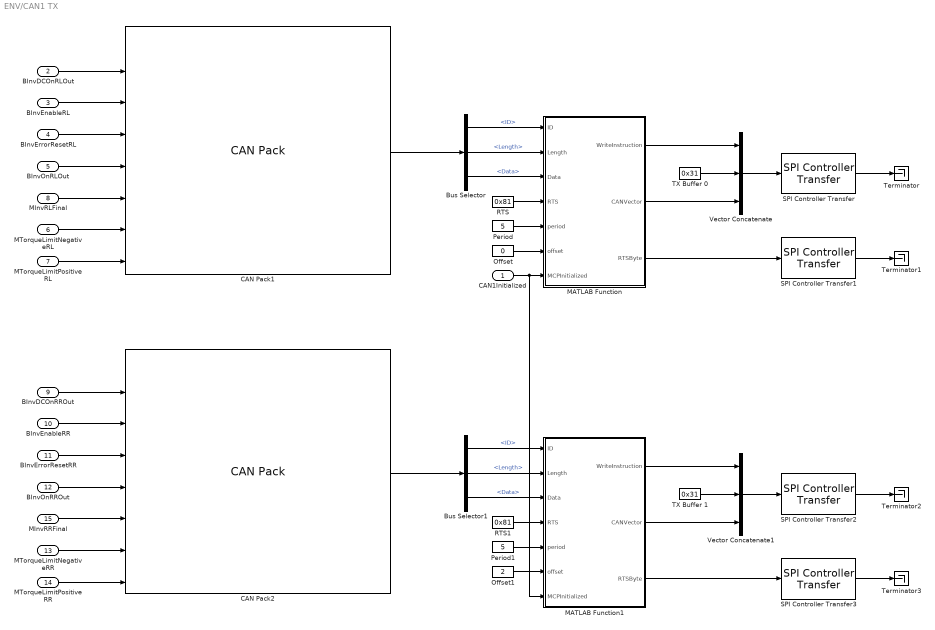
== system ENV/CAN1 TX ==
  CAN1Initialized : Inport
  BInvDCOnRLOut : Inport  Port=2
  BInvEnableRL : Inport  Port=3
  BInvErrorResetRL : Inport  Port=4
  BInvOnRLOut : Inport  Port=5
  MTorqueLimitNegativeRL : Inport  Port=6
  MTorqueLimitPositiveRL : Inport  Port=7
  MInvRLFinal : Inport  Port=8
  BInvDCOnRROut : Inport  Port=9
  BInvEnableRR : Inport  Port=10
  BInvErrorResetRR : Inport  Port=11
  BInvOnRROut : Inport  Port=12
  MTorqueLimitNegativeRR : Inport  Port=13
  MTorqueLimitPositiveRR : Inport  Port=14
  MInvRRFinal : Inport  Port=15
  Bus Selector : BusSelector  OutputSignals=ID,Length,Data
  Bus Selector1 : BusSelector  OutputSignals=ID,Length,Data
  CAN Pack1 : canmsglib/CAN Pack  CANdbFile=C:\Users\Will\Desktop\OBR\Embedded\VCUSTM32\Controls\CAN\Inverters\26.06.18_CAN1.dbc  MsgList=INV1_Receive_1  MsgName=INV1_Receive_1  MsgIDType=Standard (11-bit identifier)  MsgIdentifier=388  CANIDInput=off  MsgLength=8  Remote=off  ApplyMinMax=off  BusOutput=on  SignalInfo={'AMK_bReserve','12','8','LE','signed','Standard','0','1','0','-128','127';'BInvDCOnRLOut','9','1','LE','unsigned','Standard','0','1','0','0','1';'BInvEnableRL','10','1','LE','unsigned','Standard','0','1','0','0','1';'BInvErrorResetRL','11','1','LE','unsigned','Standard','0','1','0','0','1';'BInvOnRLOut','8','1','LE','unsigned','Standard','0','1','0','0','1';'MInvRLFinal','16','16','LE','signed','Standard','0','0.1','0','-3276.8','3276.7';'MTorqueLimitNegativeRL','48','16','LE','signed','Standard','0','0.1','0','-3276.8','3276.7';'MTorqueLimitPositiveRL','32','16','LE','signed','Standard','0','0.1','0','-3276.8','3276.7'}
      settings: LibrarySourceBlock=stmutilitieslib/CAN Pack  DataFormat=CANdb specified signals
  CAN Pack2 : canmsglib/CAN Pack  CANdbFile=C:\Users\Will\Desktop\OBR\Embedded\VCUSTM32\Controls\CAN\Inverters\26.06.18_CAN1.dbc  MsgList=INV3_Receive_1  MsgName=INV3_Receive_1  MsgIDType=Standard (11-bit identifier)  MsgIdentifier=389  CANIDInput=off  MsgLength=8  Remote=off  ApplyMinMax=off  BusOutput=on  SignalInfo={'AMK_bReserve','12','8','LE','signed','Standard','0','1','0','-128','127';'BInvDCOnRROut','9','1','LE','unsigned','Standard','0','1','0','0','1';'BInvEnableRR','10','1','LE','unsigned','Standard','0','1','0','0','1';'BInvErrorResetRR','11','1','LE','unsigned','Standard','0','1','0','0','1';'BInvOnRROut','8','1','LE','unsigned','Standard','0','1','0','0','1';'MInvRRFinal','16','16','LE','signed','Standard','0','0.1','0','-3276.8','3276.7';'MTorqueLimitNegativeRR','48','16','LE','signed','Standard','0','0.1','0','-3276.8','3276.7';'MTorqueLimitPositiveRR','32','16','LE','signed','Standard','0','0.1','0','-3276.8','3276.7'}
      settings: LibrarySourceBlock=stmutilitieslib/CAN Pack  DataFormat=CANdb specified signals
  MATLAB Function : MATLAB Function  TreatAsAtomicUnit=on
  MATLAB Function1 : MATLAB Function  TreatAsAtomicUnit=on
  Offset : Constant  Value=0  OutDataTypeStr=uint16  SampleTime=-1
  Offset1 : Constant  Value=2  OutDataTypeStr=uint16  SampleTime=-1
  Period : Constant  Value=5  OutDataTypeStr=uint16  SampleTime=-1
  Period1 : Constant  Value=5  OutDataTypeStr=uint16  SampleTime=-1
  RTS : Constant  Value=0x81  OutDataTypeStr=uint8  SampleTime=-1
  RTS1 : Constant  Value=0x81  OutDataTypeStr=uint8  SampleTime=-1
  SPI Controller Transfer : stm32blockslib/SPI Controller Transfer  Priority=1  SPIModuleSelect=SPI1  ClockPolarity=Low  ClockPhase=1 Edge  SPIModule=uint32(0)  Mode=Master  BusSpeed=uint32(1000000)  FirstBitToTransfer=Most significant bit (MSB)  ClockMode=0  BlockFunction=Transfer  EnableRegisterAddress=off  RegisterAddress=0  OutputDataType=uint8  OutputDataLength=1  OutputStatus=off  BlockingMode=off  Timeout=0.01  DataBits=8  UseCustomSSPin=Explicit GPIO calls  ActiveLowSSPin=Active low  Port_Select=GPIOB  Pin=1
      settings: LibrarySourceBlock=stm32h7xxblockslib/SPI Controller Transfer
  SPI Controller Transfer1 : stm32blockslib/SPI Controller Transfer  Priority=2  SPIModuleSelect=SPI1  ClockPolarity=Low  ClockPhase=1 Edge  SPIModule=uint32(0)  Mode=Master  BusSpeed=uint32(1000000)  FirstBitToTransfer=Most significant bit (MSB)  ClockMode=0  BlockFunction=Transfer  EnableRegisterAddress=off  RegisterAddress=0  OutputDataType=uint8  OutputDataLength=1  OutputStatus=off  BlockingMode=off  Timeout=0.01  DataBits=8  UseCustomSSPin=Explicit GPIO calls  ActiveLowSSPin=Active low  Port_Select=GPIOB  Pin=1
      settings: LibrarySourceBlock=stm32h7xxblockslib/SPI Controller Transfer
  SPI Controller Transfer2 : stm32blockslib/SPI Controller Transfer  Priority=1  SPIModuleSelect=SPI1  ClockPolarity=Low  ClockPhase=1 Edge  SPIModule=uint32(0)  Mode=Master  BusSpeed=uint32(1000000)  FirstBitToTransfer=Most significant bit (MSB)  ClockMode=0  BlockFunction=Transfer  EnableRegisterAddress=off  RegisterAddress=0  OutputDataType=uint8  OutputDataLength=1  OutputStatus=off  BlockingMode=off  Timeout=0.01  DataBits=8  UseCustomSSPin=Explicit GPIO calls  ActiveLowSSPin=Active low  Port_Select=GPIOB  Pin=1
      settings: LibrarySourceBlock=stm32h7xxblockslib/SPI Controller Transfer
  SPI Controller Transfer3 : stm32blockslib/SPI Controller Transfer  Priority=2  SPIModuleSelect=SPI1  ClockPolarity=Low  ClockPhase=1 Edge  SPIModule=uint32(0)  Mode=Master  BusSpeed=uint32(1000000)  FirstBitToTransfer=Most significant bit (MSB)  ClockMode=0  BlockFunction=Transfer  EnableRegisterAddress=off  RegisterAddress=0  OutputDataType=uint8  OutputDataLength=1  OutputStatus=off  BlockingMode=off  Timeout=0.01  DataBits=8  UseCustomSSPin=Explicit GPIO calls  ActiveLowSSPin=Active low  Port_Select=GPIOB  Pin=1
      settings: LibrarySourceBlock=stm32h7xxblockslib/SPI Controller Transfer
  TX Buffer 0 : Constant  Value=0x31  OutDataTypeStr=uint8  SampleTime=-1
  TX Buffer 1 : Constant  Value=0x31  OutDataTypeStr=uint8  SampleTime=-1
  Terminator{,1..3} (4 alike) : Terminator
  Vector Concatenate : Concatenate  NumInputs=3
  Vector Concatenate1 : Concatenate  NumInputs=3
  wires:
  SPI Controller Transfer/1 -> Terminator/1
  MATLAB Function/1(WriteInstruction) -> Vector Concatenate/1
  RTS/1 -> MATLAB Function/4(RTS)
  MATLAB Function/2(CANVector) -> Vector Concatenate/3
  SPI Controller Transfer1/1 -> Terminator1/1
  Bus Selector/1 -> MATLAB Function/1(ID)  "<ID>"
  Vector Concatenate/1 -> SPI Controller Transfer/1
  TX Buffer 0/1 -> Vector Concatenate/2
  MATLAB Function/3(RTSByte) -> SPI Controller Transfer1/1
  Bus Selector/2 -> MATLAB Function/2(Length)  "<Length>"
  Bus Selector/3 -> MATLAB Function/3(Data)  "<Data>"
  CAN Pack1/1 -> Bus Selector/1
  Period/1 -> MATLAB Function/5(period)
  Offset/1 -> MATLAB Function/6(offset)
  BInvEnableRL/1 -> CAN Pack1/3
  BInvErrorResetRL/1 -> CAN Pack1/4
  BInvDCOnRLOut/1 -> CAN Pack1/2
  SPI Controller Transfer2/1 -> Terminator2/1
  SPI Controller Transfer3/1 -> Terminator3/1
  RTS1/1 -> MATLAB Function1/4(RTS)
  MATLAB Function1/2(CANVector) -> Vector Concatenate1/3
  Bus Selector1/3 -> MATLAB Function1/3(Data)  "<Data>"
  Period1/1 -> MATLAB Function1/5(period)
  Bus Selector1/2 -> MATLAB Function1/2(Length)  "<Length>"
  Offset1/1 -> MATLAB Function1/6(offset)
  CAN Pack2/1 -> Bus Selector1/1
  Bus Selector1/1 -> MATLAB Function1/1(ID)  "<ID>"
  MATLAB Function1/3(RTSByte) -> SPI Controller Transfer3/1
  Vector Concatenate1/1 -> SPI Controller Transfer2/1
  MATLAB Function1/1(WriteInstruction) -> Vector Concatenate1/1
  TX Buffer 1/1 -> Vector Concatenate1/2
  CAN1Initialized/1 -> MATLAB Function/7(MCPInitialized), MATLAB Function1/7(MCPInitialized)
  BInvOnRLOut/1 -> CAN Pack1/5
  MInvRLFinal/1 -> CAN Pack1/6
  MTorqueLimitNegativeRL/1 -> CAN Pack1/7
  MTorqueLimitPositiveRL/1 -> CAN Pack1/8
  MInvRRFinal/1 -> CAN Pack2/6
  BInvErrorResetRR/1 -> CAN Pack2/4
  BInvOnRROut/1 -> CAN Pack2/5
  BInvEnableRR/1 -> CAN Pack2/3
  BInvDCOnRROut/1 -> CAN Pack2/2
  MTorqueLimitPositiveRR/1 -> CAN Pack2/8
  MTorqueLimitNegativeRR/1 -> CAN Pack2/7
